simulink model "untitled"  (R2013a)
settings: Solver=ode3  StartTime=0.0  StopTime=0.6  FixedStep=0.001  RelTol=1e-3
settings Model: Creator=Huy Hung  LastModifiedBy=Sion

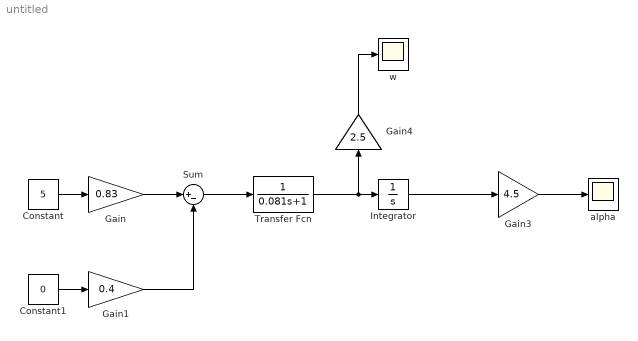
== system untitled ==
  Constant : Constant  Value=5
  Constant1 : Constant  Value=0
  Gain : Gain  Gain=0.83
  Gain1 : Gain  Gain=0.4
  Gain3 : Gain  Gain=4.5
  Gain4 : Gain  Gain=2.5
  Integrator : Integrator
  Sum : Sum  Inputs=|+-
  Transfer Fcn : TransferFcn  Denominator=[0.081 1]
  "alpha " : Scope
      settings: SaveName=alpha
  w : Scope
      settings: SaveName=w
  wires:
  Constant/1 -> Gain/1
  Transfer Fcn/1 -> Integrator/1, Gain4/1
  Constant1/1 -> Gain1/1
  Gain1/1 -> Sum/2
  Gain/1 -> Sum/1
  Sum/1 -> Transfer Fcn/1
  Gain4/1 -> w/1
  Integrator/1 -> Gain3/1
  Gain3/1 -> "alpha "/1
